simulink model "AVS_RS_SIMULINK_FIELDS_v11"  (R2020b)
settings: Solver=VariableStepAuto  StartTime=0.0  StopTime=100000  RelTol=1e-3
values from neighbouring files (symbols this model uses):
  a_s = 2    [start_SIMULINK_SIMULATION_loop.m]    (also in start_SIMULINK_SIMULATION_single.m = 1.5)
  d_between_racks = 0.5    [start_SIMULINK_SIMULATION_loop.m]    (also in start_SIMULINK_SIMULATION_single.m)
  d_first_rack = 1.5    [start_SIMULINK_SIMULATION_loop.m]    (also in start_SIMULINK_SIMULATION_single.m)
  loading_unloading_times = [4.5, 5.5, 6.5, 7.5, 8.5, 9.5]    [start_SIMULINK_SIMULATION_single.m]
  relocating_strategy = 2    [start_MATLAB_SIMULATION_loop.m]    (also in start_MATLAB_SIMULATION_single.m; start_SIMULINK_SIMULATION_single.m; states.m)
  storing_strategy = 3    [start_MATLAB_SIMULATION_loop.m]    (also in start_MATLAB_SIMULATION_single.m = 2; start_SIMULINK_SIMULATION_single.m = 2; states.m = 1)
  v_max_s = 3    [start_SIMULINK_SIMULATION_loop.m]    (also in start_SIMULINK_SIMULATION_single.m = 1.5)
  WAREHOUSE = fill_the_warehouse_1_tier(depth,racks,sides,fill)    [start_MATLAB_SIMULATION_loop.m]    (also in start_MATLAB_SIMULATION_single.m = fill_the_warehouse(depth,racks,sides,tiers,fill); start_SIMULINK_SIMULATION_loop.m = fill_the_warehouse_1_tier(depth,racks,sides,fill_alpha); start_SIMULINK_SIMULATION_single.m = fill_the_warehouse_1_tier(depth, racks, sides, fill_alpha); states.m)
undefined symbols (not defined in the file or in its folder): m, n
settings Model: PacingRate=5  Creator=Lab  LastModifiedBy=Jakob

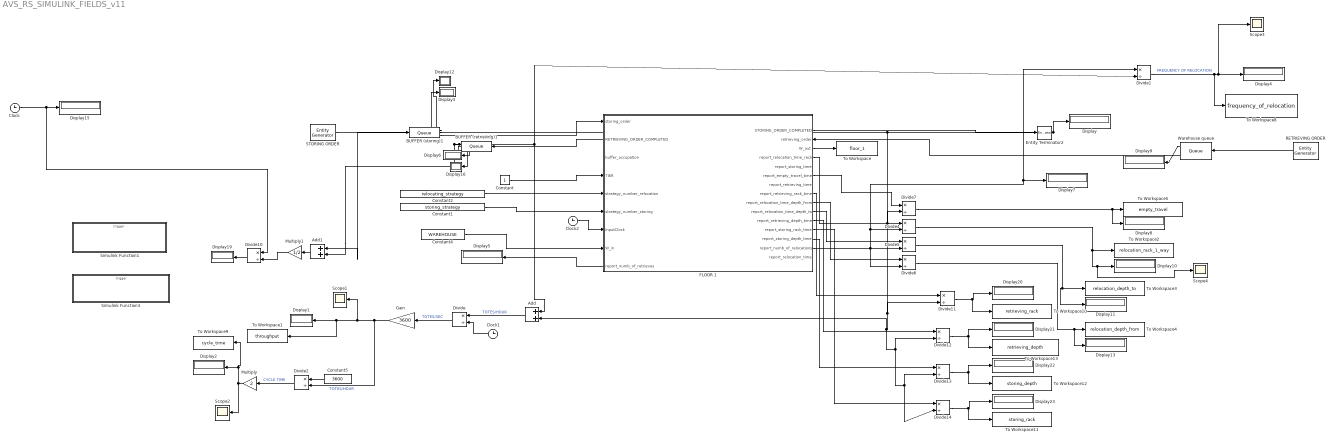
== system AVS_RS_SIMULINK_FIELDS_v11 ==
  Add : Sum
  Add1 : Sum
  BUFFER (retrieving)1 : Queue  InputPortMessageModes=m  OutputPortMessageModes=n,n,m  NumberEntitiesDeparted=on  NumberEntitiesInBlock=on
      settings: OutputPortMap=o0,o1,o5
  BUFFER (storing)1 : Queue  InputPortMessageModes=m  OutputPortMessageModes=n,n,m  NumberEntitiesDeparted=on  NumberEntitiesInBlock=on
      settings: OutputPortMap=o0,o1,o5
  Clock : Clock
  Clock1 : Clock
  Clock2 : Clock
  Constant : Constant
  Constant1 : Constant  Value=storing_strategy
  Constant2 : Constant  Value=relocating_strategy
  Constant4 : Constant  Value=WAREHOUSE
  Constant5 : Constant  Value=3600
  Display{,1..13,15..16,19..23} (21 alike) : Display
  Divide{,1..2,4..7,10..14} (12 alike) : Product  Inputs=*/
  Entity Terminator2 : EntityTerminator  InputPortMessageModes=m  NumberEntitiesArrived=on
      settings: OutputPortMap=o0
  FLOOR 1 : Stateflow chart  TreatAsAtomicUnit=on
      settings: PortSchema="{\"entries\":[{\"content\":{\"sides\":[{\"content\":{\"connectorIds\":[\"In1\",\"Out3\",\"In4\",\"In5\",\"In6\",\"In7\",\"In8\",\"In2\",\"Out5\"]},\"type\":\"ConnectorPlacement.EquallySpacedRectSide\",\"uuid\":\"b175febc-7f07-4c73-ae92-3b584758dc21\"},{\"content\":{\"connectorIds\":[\"Out1\",\"In3\",\"Out2\",\"Out7\",\"Out8\",\"Out9\",\"Out10\",\"Out14\",\"Out15\",\"Out16\",\"Out11\",\"Out12\",\"Out13\",\"Out4\",\"Out6\"],\"side\":\"RIGHT\"},\"type\":\"ConnectorPlacement.EquallySpacedRectSide\",\"uuid\":\"34175d97-0745-47d9-92aa-761f07cc1cff\"},{\"content\":{\"connectorIds\":[],\"side\":\"TOP\"},\"type\":\"ConnectorPlacement.EquallySpacedRectSide\",\"uuid\":\"f23de919-4082-4448-95b1-60435026244c\"}]},\"type\":\"ConnectorPlacement.EquallySpacedConnector\",\"uuid\":\"d04e0a1a-0e62-411a-89ea-55346d2e3dbb\"}],\"packageUris\":[\"http://schema.mathworks.com/mf0/Connector/19700101\"],\"version\":\"1.0\"}"
  Gain : Gain  Gain=3600
  Multiply : Gain  Gain=2
  Multiply1 : Gain  Gain=1/2
  RETRIEVING ORDER : EntityGenerator  OutputPortMessageModes=m  GenerateEntityAtSimulationStart=off  GenerateAction=|  EntityType=Bus object  EntityTypeName=Task
      | % [out_d,out_r,out_s,out_t, out_SKU] = find_SKU_position()
      | % 
      | % entity.START_TIER = out_t
      | % entity.START_DEPTH = out_d
      | % entity.START_RACK = out_r
      | % entity.START_SIDE = out_s
      | % 
      | % 
      | entity.GOAL_TIER = 1;
      | entity.GOAL_DEPTH = 0;
      | entity.GOAL_RACK = 0;
      | entity.GOAL_SIDE = 0;
      | 
      | 
      | 
      | 
      | %Pattern: Repeating Sequence
      | 
      | entity.SKU_ID = -1;
      | entity.TYPE = 1;
  STORING ORDER : EntityGenerator  OutputPortMessageModes=m  GenerateAction=|  EntityType=Bus object  EntityTypeName=Task
      | entity.START_TIER = 0;
      | entity.START_DEPTH = 0;
      | entity.START_RACK = 0;
      | entity.START_SIDE = 0;
      | 
      | 
      | % Pattern: Repeating Sequence
      | 
      | persistent idx;
      | if isempty(idx)
      |     idx = max(max(max(WAREHOUSE)))+1;
      | else 
      |     idx = idx + 1;
      | end
      | 
      | entity.SKU_ID = idx;
      | entity.TYPE = 0;
  Scope{1..4} (4 alike) : Scope
  Simulink Function1 : Subsystem  TreatAsAtomicUnit=on
  Simulink Function3 : Subsystem  TreatAsAtomicUnit=on
  To Workspace : ToWorkspace  VariableName=floor_1  SaveFormat=Timeseries  SampleTime=-1
  To Workspace1 : ToWorkspace  VariableName=throughput  SaveFormat=Timeseries  SampleTime=-1
  To Workspace10 : ToWorkspace  VariableName=retrieving_rack  SaveFormat=Timeseries  SampleTime=-1
  To Workspace11 : ToWorkspace  VariableName=storing_rack  SaveFormat=Timeseries  SampleTime=-1
  To Workspace12 : ToWorkspace  VariableName=storing_depth  SaveFormat=Timeseries  SampleTime=-1
  To Workspace13 : ToWorkspace  VariableName=retrieving_depth  SaveFormat=Timeseries  SampleTime=-1
  To Workspace2 : ToWorkspace  VariableName=relocation_rack_1_way  SaveFormat=Timeseries  SampleTime=-1
  To Workspace3 : ToWorkspace  VariableName=relocation_depth_to  SaveFormat=Timeseries  SampleTime=-1
  To Workspace4 : ToWorkspace  VariableName=relocation_depth_from  SaveFormat=Timeseries  SampleTime=-1
  To Workspace5 : ToWorkspace  VariableName=empty_travel  SaveFormat=Timeseries  SampleTime=-1
  To Workspace8 : ToWorkspace  VariableName=frequency_of_relocation  SaveFormat=Timeseries  SampleTime=-1
  To Workspace9 : ToWorkspace  VariableName=cycle_time  SaveFormat=Timeseries  SampleTime=-1
  Warehouse queue : Queue  InputPortMessageModes=m  OutputPortMessageModes=n,m  NumberEntitiesDeparted=on
      settings: OutputPortMap=o0,o5
  wires:
  STORING ORDER/1 -> BUFFER (storing)1/1
  FLOOR 1/1(STORING_ORDER_COMPLETED) -> Entity Terminator2/1
  FLOOR 1/2(W_out) -> To Workspace/1
  RETRIEVING ORDER/1 -> Warehouse queue/1
  BUFFER (storing)1/3 -> FLOOR 1/1(storing_order)
  BUFFER (storing)1/2 -> Display12/1
  FLOOR 1/4(report_numb_of_relocations) -> Divide6/2, Divide5/2, Display7/1, Divide1/1, Divide4/2
  Warehouse queue/2 -> FLOOR 1/3(retrieving_order)
  Warehouse queue/1 -> Display9/1
  Clock/1 -> Divide10/1, Display15/1
  FLOOR 1/3(RETRIEVING_ORDER_COMPLETED) -> BUFFER (retrieving)1/1
  BUFFER (retrieving)1/2 -> Display16/1
  BUFFER (storing)1/1 -> Display3/1
  Constant4/1 -> FLOOR 1/2(W_in)
  Constant/1 -> FLOOR 1/5(TIER)
  Divide2/1 -> Multiply/1  "CYCLE TIME"
  Divide/1 -> Gain/1  "TOTES/SEC"
  Constant5/1 -> Divide2/1
  Gain/1 -> Divide2/2, To Workspace1/1, Display1/1, Scope1/1  "TOTES/HOUR"
  BUFFER (retrieving)1/1 -> Add1/2, Display6/1, Divide1/2, Add/1
  Multiply/1 -> Scope2/1, To Workspace9/1, Display2/1
  Entity Terminator2/1 -> Add1/1, Divide7/2, Divide14/2, Divide13/2, Divide12/2, Add/2, Divide11/2, Display/1
  Clock1/1 -> Divide/2
  Divide1/1 -> Display4/1, Scope3/1, To Workspace8/1  "FREQUENCY OF RELOCATION"
  Constant1/1 -> FLOOR 1/7(strategy_number_storing)
  Constant2/1 -> FLOOR 1/6(strategy_number_relocation)
  Add/1 -> Divide/1  "TOTES/HOUR"
  Clock2/1 -> FLOOR 1/8(InputClock)
  FLOOR 1/5(report_numb_of_retrieves) -> Display5/1
  FLOOR 1/7(report_relocation_time_rack) -> Divide4/1
  FLOOR 1/16(report_relocation_time_depth_to) -> Divide5/1
  Divide4/1 -> Scope4/1, Display10/1, To Workspace2/1
  Divide5/1 -> Display11/1, To Workspace3/1
  Divide6/1 -> To Workspace4/1, Display13/1
  Add1/1 -> Multiply1/1
  Multiply1/1 -> Divide10/2
  Divide10/1 -> Display19/1
  Divide11/1 -> To Workspace10/1, Display20/1
  Divide12/1 -> Display21/1, To Workspace13/1
  Divide13/1 -> Display22/1, To Workspace12/1
  Divide14/1 -> To Workspace11/1, Display23/1
  FLOOR 1/14(report_retrieving_rack_time) -> Divide11/1
  FLOOR 1/11(report_retrieving_depth_time) -> Divide12/1
  FLOOR 1/12(report_storing_rack_time) -> Divide14/1
  FLOOR 1/13(report_storing_depth_time) -> Divide13/1
  Divide7/1 -> Display8/1, To Workspace5/1
  FLOOR 1/9(report_empty_travel_time) -> Divide7/1
  FLOOR 1/15(report_relocation_time_depth_from) -> Divide6/1

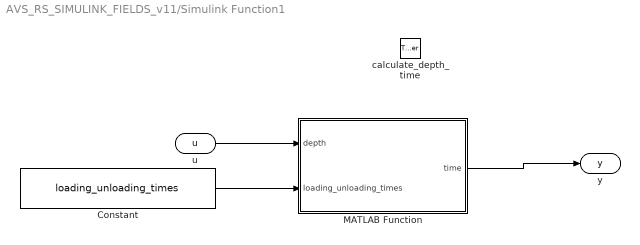
== system AVS_RS_SIMULINK_FIELDS_v11/Simulink Function1 ==
  calculate_depth_time : TriggerPort  TriggerType=function-call  IsSimulinkFunction=on  FunctionName=calculate_depth_time  FunctionVisibility=scoped  VariantControl=(inherit)
  Constant : Constant  Value=loading_unloading_times
  MATLAB Function : MATLAB Function  TreatAsAtomicUnit=on
  u : ArgIn  DisableCoverage=on  ArgumentName=u
  y : ArgOut  DisableCoverage=on  ArgumentName=y
  wires:
  u/1 -> MATLAB Function/1(depth)
  MATLAB Function/1(time) -> y/1
  Constant/1 -> MATLAB Function/2(loading_unloading_times)

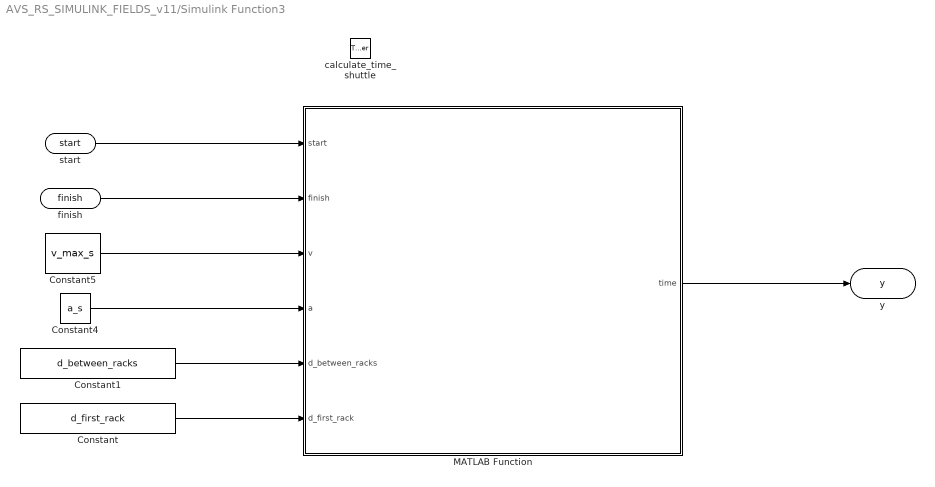
== system AVS_RS_SIMULINK_FIELDS_v11/Simulink Function3 ==
  calculate_time_shuttle : TriggerPort  TriggerType=function-call  IsSimulinkFunction=on  FunctionName=calculate_time_shuttle  FunctionVisibility=scoped  VariantControl=(inherit)
  Constant : Constant  Value=d_first_rack
  Constant1 : Constant  Value=d_between_racks
  Constant4 : Constant  Value=a_s
  Constant5 : Constant  Value=v_max_s
  MATLAB Function : MATLAB Function  TreatAsAtomicUnit=on
  start : ArgIn  DisableCoverage=on  ArgumentName=start
  finish : ArgIn  DisableCoverage=on  Port=2  ArgumentName=finish
  y : ArgOut  DisableCoverage=on  ArgumentName=y
  wires:
  Constant5/1 -> MATLAB Function/3(v)
  start/1 -> MATLAB Function/1(start)
  finish/1 -> MATLAB Function/2(finish)
  MATLAB Function/1(time) -> y/1
  Constant4/1 -> MATLAB Function/4(a)
  Constant1/1 -> MATLAB Function/5(d_between_racks)
  Constant/1 -> MATLAB Function/6(d_first_rack)

== stateflow chart AVS_RS_SIMULINK_FIELDS_v11/FLOOR 1 ==
  settings: enableNonTerminalStates=1
  state STORING_CYLCE [group]
    state CHECK_FOR_RETRIEVAL
    state STORING_COMPLETED
      entry:
      W(goal_d, goal_r, goal_s) =Vehicle_Occupation.data.SKU_ID;
      W_out = W;
      report_storing_time =report_storing_time+ calculate_depth_time(goal_d) + ...
      calculate_depth_time(1) + TRAVEL_TIME_RACK;
      %STORING_ORDER_COMPLETED.data = Vehicle_Occupation.data
    state STORING_RETURNING_DEPTH
      entry:
      TRAVEL_TIME_DEPTH = calculate_depth_time(goal_d);
      report_storing_depth_time = report_storing_depth_time + goal_d;
    state STORING_ARIEVED
    state LOADING_SKU
      entry:
      [goal_d, goal_r, goal_s] = STORING_strategy(strategy_number_storing,W);
      start_d = 0; start_r=0; start_t=tier; start_s=0;
      TRAVEL_TIME_RACK = calculate_time_shuttle(start_r, goal_r);
      report_storing_rack_time = report_storing_rack_time + goal_r;
      TRAVEL_TIME_DEPTH = calculate_depth_time(1);
      Vehicle_Occupation.data = storing_order.data;
      forward(storing_order, Vehicle_Occupation);
    state STORING_ORDER_START
    state Idle
    CHECK_FOR_RETRIEVAL -> Idle [order 2] : after(TRAVEL_TIME_RACK,sec)
    STORING_COMPLETED -> CHECK_FOR_RETRIEVAL : Vehicle_Occupation{forward(Vehicle_Occupation, STORING_ORDER_COMPLETED)}
    STORING_RETURNING_DEPTH -> STORING_COMPLETED : after(TRAVEL_TIME_DEPTH, sec)
    STORING_ARIEVED -> STORING_RETURNING_DEPTH : after(0,sec)
    STORING_ORDER_START -> STORING_ARIEVED : after(TRAVEL_TIME_RACK, sec)
    (default) -> Idle : {W = W_in(:,:,:,TIER);
        | tier =TIER;
        | number_of_relocations = 0;
        | number_of_retrieves = 0;
        | report_numb_of_retrieves = 0;
        | BUFFER_LIMIT = 1;
        | report_relocation_time = 0;
        | report_relocation_time_rack = 0;
        | report_relocation_time_depth_from = 0;
        | report_relocation_time_depth_to = 0;
        | report_storing_time = 0;
        | report_empty_travel_time=0;
        | report_retrieving_time = 0;
        | current_relocation_time = 0;
        | current_relocation_time_rack = 0;
        | current_relocation_time_depth_to = 0;
        | current_relocation_time_depth_from = 0;
        | report_storing_depth_time = 0;
        | report_storing_rack_time = 0;
        | report_retrieving_rack_time = 0;
        | report_retrieving_depth_time = 0;}
    LOADING_SKU -> STORING_ORDER_START : after(TRAVEL_TIME_DEPTH, sec)
    Idle -> LOADING_SKU [order 1] : storing_order
  state DCC [group]
    state DUAL_COMMAND_CYCLE
      entry:
      target_SKU = select_random_SKU_3D(W);
      start_r = goal_r;
      [goal_d, goal_r, goal_s] = find_SKU_position(target_SKU, W);
      %assign attributes to order
      retrieving_order.data.START_DEPTH = goal_d;
      retrieving_order.data.START_TIER = tier;
      %retrieving_order.data.START_SIDE
      retrieving_order.data.START_RACK= goal_r;
      retrieving_order.data.SKU_ID = target_SKU;
      TRAVEL_TIME_RACK = calculate_time_shuttle(start_r, goal_r);
      forward(retrieving_order, Vehicle_Occupation);
      report_empty_travel_time = report_empty_travel_time + abs(goal_r-start_r);
    state RELOCATION_TEST
      entry:
      %relocation test
      [relo_d, relo_r, relo_s, relo_necessity] = relocation_necessity_test(W, target_SKU);
      report_relocation_time_depth_from = report_relocation_time_depth_from + current_relocation_time_depth_from;
      current_relocation_time_depth_from = 0;
      report_relocation_time_rack = report_relocation_time_rack + current_relocation_time_rack;
      current_relocation_time_rack = 0;
      report_relocation_time_depth_to = report_relocation_time_depth_to + current_relocation_time_depth_to;
      current_relocation_time_depth_to = 0;
    state RETRIEVING_ARIVED_DCC_
      entry:
      TRAVEL_TIME_DEPTH = calculate_depth_time(goal_d);
      report_retrieving_depth_time = report_retrieving_depth_time + goal_d ;
    DUAL_COMMAND_CYCLE -> DCC.RELOCATION_TEST : after(TRAVEL_TIME_RACK, sec)
    DCC.RELOCATION_TEST -> (junction 163) : after(0, sec)
    (junction 163) -> RETRIEVING_ARIVED_DCC_ [order 2]
  state RELOCATION CYCLE DCC [group]
    state RELOCATION_END
      entry:
      current_relocation_time_depth_to = current_relocation_time_depth_to + new_d ;
    state RELOCATION_CYCLE_TRAVEL2
      entry:
      TRAVEL_TIME_RACK = calculate_time_shuttle(new_r, goal_r);
    state RELOCATION_CYCLE_TRAVEL1
      entry:
      W(new_d, new_r, new_s) = RELOCATING_SKU;
    state RELOCATION_CYCLE_TRAVEL
      entry:
      current_relocation_time_rack = abs(relo_r-new_r);
    state RELOCATION_CYCLE_SKU_LOADED
    state RELOCATION_CYCLE_SKU_LOADED1
      entry:
      %insert relocation strategy
      [new_d, new_r, new_s] = RELOCATION_strategy(strategy_number_relocation,W, relo_r, relo_s);
      TRAVEL_TIME_RACK = calculate_time_shuttle(relo_r, new_r);
      TRAVEL_TIME_DEPTH = calculate_depth_time(new_d);
      W(relo_d, relo_r, relo_s) = 0;
    state RELOCATION_CYCLE_START
      entry:
      TRAVEL_TIME_DEPTH = calculate_depth_time(relo_d);
      RELOCATING_SKU = W(relo_d, relo_r, relo_s);
      number_of_relocations = number_of_relocations +1;
      report_numb_of_relocations = number_of_relocations;
      start_relocation_time = InputClock();
      current_relocation_time_depth_from = relo_d;
    RELOCATION.RELOCATION_CYCLE_TRAVEL -> RELOCATION.RELOCATION_CYCLE_TRAVEL1 : after(TRAVEL_TIME_DEPTH , sec)
    RELOCATION.RELOCATION_CYCLE_TRAVEL1 -> RELOCATION.RELOCATION_CYCLE_TRAVEL2 : after(0, sec)
    RELOCATION.RELOCATION_CYCLE_TRAVEL2 -> RELOCATION_END : after(TRAVEL_TIME_RACK, sec)
    RELOCATION.RELOCATION_CYCLE_SKU_LOADED1 -> RELOCATION.RELOCATION_CYCLE_TRAVEL : after(TRAVEL_TIME_RACK,sec)
    RELOCATION.RELOCATION_CYCLE_START -> RELOCATION.RELOCATION_CYCLE_SKU_LOADED : after(TRAVEL_TIME_DEPTH , sec)
    RELOCATION.RELOCATION_CYCLE_SKU_LOADED -> RELOCATION.RELOCATION_CYCLE_SKU_LOADED1 : after(0, sec)
  state RETRIEVING CYCLE [group]
    state RETRIEVING_ARRIVED_BACK
    state RETRIEVING_SKU_LOADED
      entry:
      W(goal_d, goal_r, goal_s) = 0;
      start_d = 0; start_r = goal_r;
      goal_d = 1; goal_r = 0; goal_s = 1;
      TRAVEL_TIME_RACK = calculate_time_shuttle(start_r, goal_r);
      report_retrieving_rack_time = report_retrieving_rack_time+ abs(start_r - goal_r);
      TRAVEL_TIME_DEPTH = calculate_depth_time(1);
      number_of_retrieves = number_of_retrieves + 1;
      report_numb_of_retrieves = number_of_retrieves;
    state RETRIEVING_COMPLETED
      entry:
      W_out = W;
    state CHECKING_BUFFER
    state RETRIEVING_ORDER
      entry:
      target_SKU = select_random_SKU_3D(W);
      start_r = 0;
      [goal_d, goal_r, goal_s] = find_SKU_position(target_SKU, W);
      %assign attributes to order
      retrieving_order.data.START_DEPTH = goal_d;
      retrieving_order.data.START_TIER = tier;
      %retrieving_order.data.START_SIDE
      retrieving_order.data.START_RACK= goal_r;
      retrieving_order.data.SKU_ID = target_SKU;
      TRAVEL_TIME_RACK = calculate_time_shuttle(start_r, goal_r);
      forward(retrieving_order, Vehicle_Occupation);
    state RELOCATION_TEST
      entry:
      %relocation test
      [relo_d, relo_r, relo_s, relo_necessity] = relocation_necessity_test(W, target_SKU);
    state RETRIEVING_ARRIEVED
    (junction 212) -> RETRIEVING_ARRIVED_BACK [order 1] : [buffer_occupation < BUFFER_LIMIT]
    RETRIEVING_SKU_LOADED -> (junction 212) : after(TRAVEL_TIME_RACK , sec)
    (junction 212) -> CHECKING_BUFFER [order 2]
    RETRIEVING_ARRIVED_BACK -> RETRIEVING_COMPLETED : after(TRAVEL_TIME_DEPTH, sec)
    (junction 209) -> RETRIEVING_ARRIVED_BACK [order 1] : [[buffer_occupation < BUFFER_LIMIT]]
    RETRIEVING_ARRIEVED -> RETRIEVING_SKU_LOADED : after(load_time, sec)
    (junction 209) -> CHECKING_BUFFER [order 2]
    CHECKING_BUFFER -> (junction 209) : after(0.01, sec)
    RETRIEVING_ORDER -> RETRIEVING.RELOCATION_TEST : after(0, sec)
    RETRIEVING.RELOCATION_TEST -> (junction 196) : after(TRAVEL_TIME_RACK, sec)
    (junction 196) -> RETRIEVING_ARRIEVED [order 2]
  state RELOCATION1 CYCLE SCC [group]
    state RELOCATION_CYCLE_START
      entry:
      TRAVEL_TIME_DEPTH = calculate_depth_time(relo_d);
      RELOCATING_SKU = W(relo_d, relo_r, relo_s)
      number_of_relocations = number_of_relocations +1
      report_numb_of_relocations = number_of_relocations
    state RELOCATION_CYCLE_SKU_LOADED
      entry:
      W(relo_d, relo_r, relo_s) = 0;
    state RELOCATION_CYCLE_SKU_LOADED1
      entry:
      %insert relocation strategy
      [new_d, new_r, new_s] = find_random_empty_slot(W)
      TRAVEL_TIME_RACK = calculate_time_shuttle(relo_r, new_r);
      TRAVEL_TIME_DEPTH = calculate_depth_time(new_d);
    state RELOCATION_CYCLE_TRAVEL2
      entry:
      TRAVEL_TIME_RACK = calculate_time_shuttle(new_r, goal_r)
    state RELOCATION_CYCLE_TRAVEL1
      entry:
      W(new_d, new_r, new_s) = RELOCATING_SKU
    state RELOCATION_CYCLE_TRAVEL
    RELOCATION1.RELOCATION_CYCLE_START -> RELOCATION1.RELOCATION_CYCLE_SKU_LOADED : after(TRAVEL_TIME_DEPTH + load_time, sec)
    RELOCATION1.RELOCATION_CYCLE_SKU_LOADED -> RELOCATION1.RELOCATION_CYCLE_SKU_LOADED1 : after(TRAVEL_TIME_DEPTH, sec)
    RELOCATION1.RELOCATION_CYCLE_SKU_LOADED1 -> RELOCATION1.RELOCATION_CYCLE_TRAVEL : after(TRAVEL_TIME_RACK,sec)
    RELOCATION1.RELOCATION_CYCLE_TRAVEL1 -> RELOCATION1.RELOCATION_CYCLE_TRAVEL2 : after(TRAVEL_TIME_DEPTH, sec)
    RELOCATION1.RELOCATION_CYCLE_TRAVEL -> RELOCATION1.RELOCATION_CYCLE_TRAVEL1 : after(TRAVEL_TIME_DEPTH + unload_time, sec)
  CHECK_FOR_RETRIEVAL -> DUAL_COMMAND_CYCLE [order 1] : retrieving_order
  RELOCATION_END -> DCC.RELOCATION_TEST : after(0,sec)
  (junction 163) -> RELOCATION.RELOCATION_CYCLE_START [order 1] : [relo_necessity == 1]
  RETRIEVING_ARIVED_DCC_ -> RETRIEVING_SKU_LOADED : after(TRAVEL_TIME_DEPTH , sec)
  Idle -> RETRIEVING_ORDER [order 2] : retrieving_order
  RETRIEVING_COMPLETED -> Idle : Vehicle_Occupation{forward(Vehicle_Occupation, RETRIEVING_ORDER_COMPLETED)}
  (junction 196) -> RELOCATION1.RELOCATION_CYCLE_START [order 1] : [relo_necessity == 1]
  RELOCATION1.RELOCATION_CYCLE_TRAVEL2 -> RETRIEVING.RELOCATION_TEST
  data: storing_order input Bus: Task; STORING_ORDER_COMPLETED output Bus: Task; unload_time constant double =0; W local; W_in input; W_out output; target_SKU local; load_time constant double =3.4; RETRIEVING_ORDER_COMPLETED output Bus: Task; retrieving_order input Bus: Task; start_d local; start_s local; start_t local; TRAVEL_TIME_DEPTH local; TRAVEL_TIME_RACK local; goal_d local; goal_r local; goal_s local; start_r local; Vehicle_Occupation local Bus: Task; tier local; relo_necessity local; relo_d local; relo_r local; relo_s local; RELOCATING_SKU local; new_d local; new_r local; new_s local; number_of_relocations local; report_numb_of_relocations output; report_numb_of_retrieves output; number_of_retrieves local; BUFFER_LIMIT local; buffer_occupation input; TIER input; strategy_number_relocation input; strategy_number_storing input; report_relocation_time output; current_relocation_time local; start_relocation_time local; InputClock input; current_relocation_time_rack local; report_relocation_time_rack output; report_storing_time output; report_empty_travel_time output; report_retrieving_time output; report_retrieving_depth_time output; report_storing_rack_time output; report_storing_depth_time output; report_retrieving_rack_time output; report_relocation_time_depth_from output; report_relocation_time_depth_to output; current_relocation_time_depth_from local; current_relocation_time_depth_to local

== matlab function AVS_RS_SIMULINK_FIELDS_v11/Simulink Function1/MATLAB Function ==
  data: depth input; time output; loading_unloading_times input
function time = fcn(depth,loading_unloading_times)

if depth < 1
    time =0;
    
elseif depth < 2
    time = loading_unloading_times(1);
elseif depth < 3
    time = loading_unloading_times(2);
elseif depth < 4
    time = loading_unloading_times(3);
elseif depth < 5
    time = loading_unloading_times(4);   
    
elseif depth < 6
    time = loading_unloading_times(5);      
    
else
    time = loading_unloading_times(6);

end

return

== matlab function AVS_RS_SIMULINK_FIELDS_v11/Simulink Function3/MATLAB Function ==
  data: start input; time output; finish input; v input; a input; d_between_racks input; d_first_rack input
function time = fcn(start, finish, v, a,d_between_racks, d_first_rack)

path = abs(finish-start) * d_between_racks;

if finish == 0 || start == 0    
    path = path + d_first_rack - d_between_racks;
    
elseif finish == start
    path = 0;   

end
    
critical_path = (v^2)/a;


if path < critical_path
    time = 2*(path/a)^0.5;
    return
    
else
    time = (path/v) + (v/a);
    return
    
end
